simulink model "dual_motor_pitch_openloop"  (R2021b)
settings: Solver=ode45  StartTime=0.0  StopTime=100  MaxStep=1e-3  RelTol=1e-6  AbsTol=1e-8
settings Model: Creator=xuan1  LastModifiedBy=xuan1

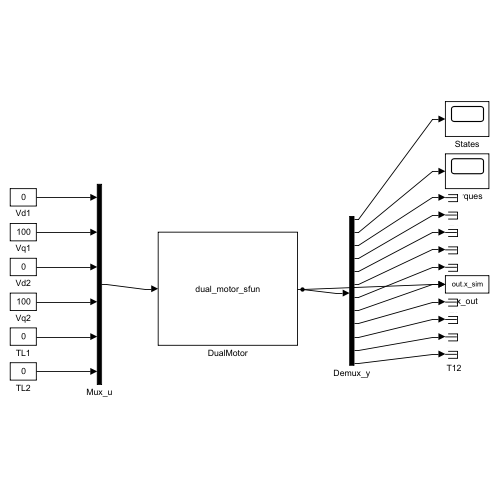
[thumbnail: Simulink's stored preview of the top-level diagram]
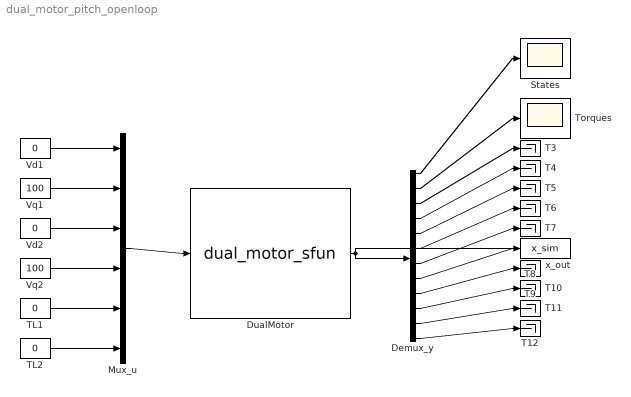
== system dual_motor_pitch_openloop ==
  Demux_y : Demux  Outputs=12
  DualMotor : S-Function  FunctionName=dual_motor_sfun  SFunctionDeploymentMode=off  EnableBusSupport=off
  Mux_u : Mux  Inputs=6
  States : Scope
  T{3..12} (10 alike) : Terminator
  TL1 : Constant  Value=0
  TL2 : Constant  Value=0
  Torques : Scope
  Vd1 : Constant  Value=0
  Vd2 : Constant  Value=0
  Vq1 : Constant  Value=100
  Vq2 : Constant  Value=100
  x_out : ToWorkspace  VariableName=x_sim  SaveFormat=Timeseries  SampleTime=-1
  wires:
  Vd1/1 -> Mux_u/1
  Vq1/1 -> Mux_u/2
  Vd2/1 -> Mux_u/3
  Vq2/1 -> Mux_u/4
  TL1/1 -> Mux_u/5
  TL2/1 -> Mux_u/6
  Mux_u/1 -> DualMotor/1
  DualMotor/1 -> Demux_y/1, x_out/1
  Demux_y/1 -> States/1
  Demux_y/2 -> Torques/1
  Demux_y/3 -> T3/1
  Demux_y/4 -> T4/1
  Demux_y/5 -> T5/1
  Demux_y/6 -> T6/1
  Demux_y/7 -> T7/1
  Demux_y/8 -> T8/1
  Demux_y/9 -> T9/1
  Demux_y/10 -> T10/1
  Demux_y/11 -> T11/1
  Demux_y/12 -> T12/1
